simulink model "position_subsystem_dob"  (R2019b)
settings: Solver=VariableStepAuto  StartTime=0.0  StopTime=100  RelTol=1e-3
values from neighbouring files (symbols this model uses):
  G__X_N = G__V_N_PX4_CL*(1/s)    [dob_design.m]
  P__X_N = MPC_XY_P    [dob_design.m]
  Q_2nd_DEM = [1 2*Q_zeta*wn wn^2]    [dob_design.m]
  Q_2nd_NUM = [0 0 1]    [dob_design.m]
undefined symbols (not defined in the file or in its folder): K, P, R
libraries: simulink x1
settings Model: Creator=henry  LastModifiedBy=henry

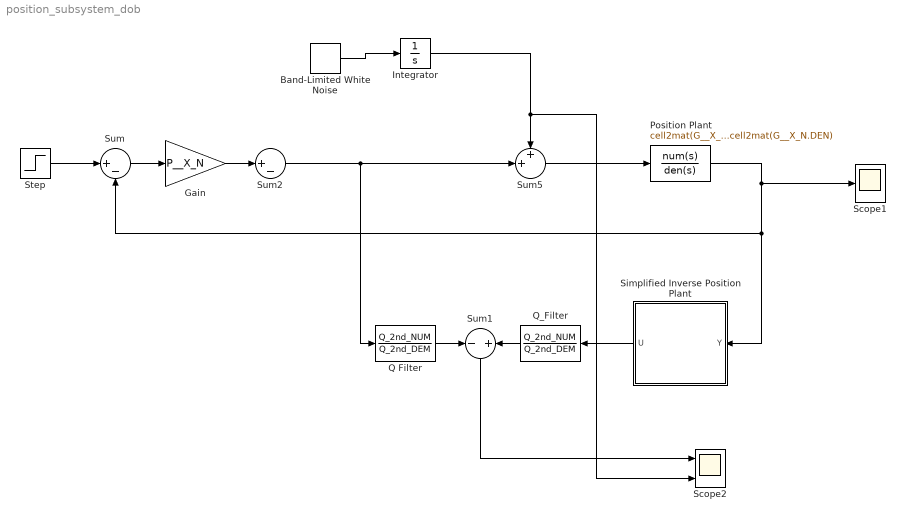
== system position_subsystem_dob ==
  Band-Limited White Noise : simulink/Sources/Band-Limited White Noise  Cov=[0.2]  Ts=0.1  seed=[23341]
  Gain : Gain  Gain=P__X_N
  Integrator : Integrator
  Position Plant : TransferFcn  Numerator=cell2mat(G__X_N.NUM)  Denominator=cell2mat(G__X_N.DEN)
  Q Filter : TransferFcn  Numerator=Q_2nd_NUM  Denominator=Q_2nd_DEM
  Q_Filter : TransferFcn  Numerator=Q_2nd_NUM  Denominator=Q_2nd_DEM
  Scope1 : Scope
  Scope2 : Scope  NumInputPorts=2
  Simplified Inverse Position Plant : Subsystem
  Step : Step  Time=2  After=0.1  SampleTime=0
  Sum : Sum  Inputs=|+-
  Sum1 : Sum  Inputs=-+
  Sum2 : Sum  Inputs=|+-
  Sum5 : Sum  Inputs=++|
  wires:
  Position Plant/1 -> Scope1/1, Simplified Inverse Position Plant/1(Y), Sum/2
  Sum/1 -> Gain/1
  Step/1 -> Sum/1
  Sum5/1 -> Position Plant/1
  Q_Filter/1 -> Sum1/2
  Q Filter/1 -> Sum1/1
  Gain/1 -> Sum2/1
  Sum2/1 -> Q Filter/1, Sum5/2
  Sum1/1 -> Scope2/1
  Simplified Inverse Position Plant/1(U) -> Q_Filter/1
  Integrator/1 -> Scope2/2, Sum5/1
  Band-Limited White Noise/1 -> Integrator/1

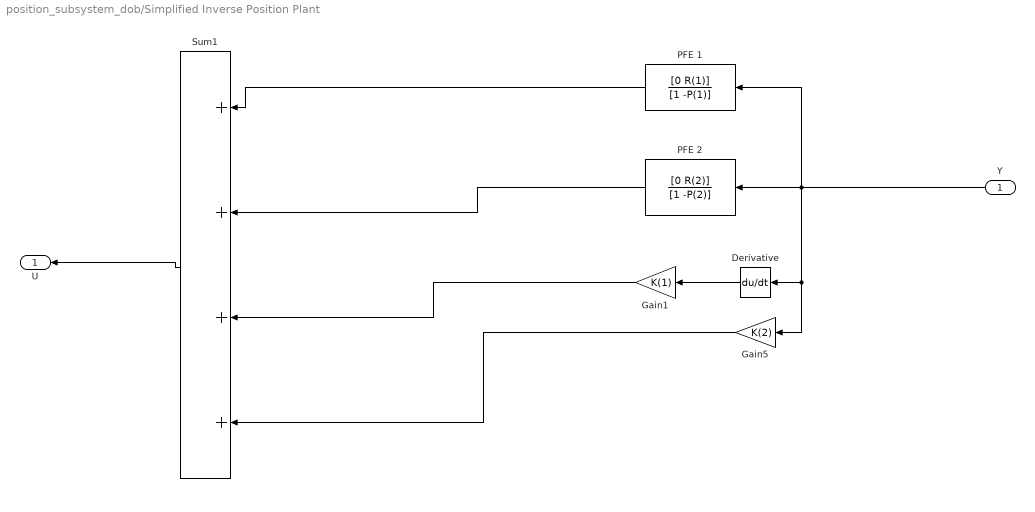
== system position_subsystem_dob/Simplified Inverse Position Plant ==
  Y : Inport
  Derivative : Derivative
  Gain1 : Gain  Gain=K(1)
  Gain5 : Gain  Gain=K(2)
  PFE 1 : TransferFcn  Numerator=[0 R(1)]  Denominator=[1 -P(1)]
  PFE 2 : TransferFcn  Numerator=[0 R(2)]  Denominator=[1 -P(2)]
  Sum1 : Sum  Inputs=++++
  U : Outport
  wires:
  Sum1/1 -> U/1
  Y/1 -> PFE 1/1, Derivative/1, Gain5/1, PFE 2/1
  Derivative/1 -> Gain1/1
  PFE 2/1 -> Sum1/2
  PFE 1/1 -> Sum1/1
  Gain1/1 -> Sum1/3
  Gain5/1 -> Sum1/4
